simulink model "rajada"  (R2016a)
settings: Solver=VariableStepAuto  StartTime=0.0  StopTime=10.0  RelTol=1e-3
values from neighbouring files (symbols this model uses):
  dt = 0.005    [main.m]
  MC = MI*CC    [main.m]
  MFT = MI*FT    [main.m]
  MFW = MI*FW    [main.m]
  MK = MI*KK    [main.m]
settings Model: Creator=Geraldo  LastModifiedBy=Geraldo

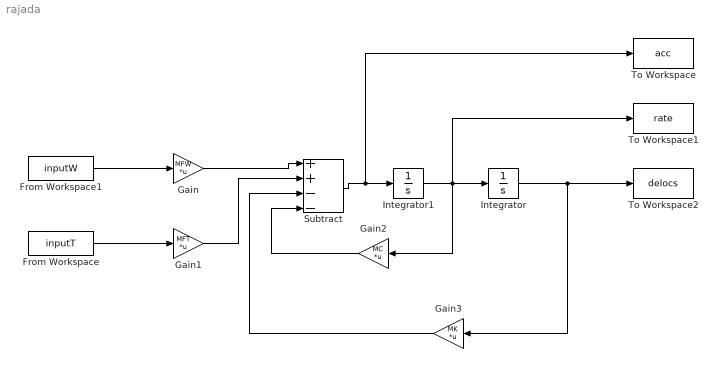
== system rajada ==
  From Workspace : FromWorkspace  VariableName=inputT  SampleTime=dt
  From Workspace1 : FromWorkspace  VariableName=inputW  SampleTime=dt
  Gain : Gain  Gain=MFW  Multiplication=Matrix(K*u)
  Gain1 : Gain  Gain=MFT  Multiplication=Matrix(K*u)
  Gain2 : Gain  Gain=MC  Multiplication=Matrix(K*u)
  Gain3 : Gain  Gain=MK  Multiplication=Matrix(K*u)
  Integrator : Integrator
  Integrator1 : Integrator
  Subtract : Sum  Inputs=++--
  To Workspace : ToWorkspace  VariableName=acc  SampleTime=dt
  To Workspace1 : ToWorkspace  VariableName=rate  SampleTime=dt
  To Workspace2 : ToWorkspace  VariableName=delocs  SampleTime=dt
  wires:
  From Workspace1/1 -> Gain/1
  Gain/1 -> Subtract/1
  From Workspace/1 -> Gain1/1
  Gain1/1 -> Subtract/2
  Integrator1/1 -> Gain2/1, To Workspace1/1, Integrator/1
  Integrator/1 -> Gain3/1, To Workspace2/1
  Gain3/1 -> Subtract/3
  Gain2/1 -> Subtract/4
  Subtract/1 -> To Workspace/1, Integrator1/1
